simulink model "rake"  (R2017b)
settings: Solver=FixedStepDiscrete  StartTime=0.0  StopTime=0.1  RelTol=1e-3
PreLoadFcn:
  | commwcdmaphlayer_init;
undefined symbols (not defined in the file or in its folder): doppler, totalBitsDelay, trBlkSetSize, tti
libraries: commwcdma_lib x7, commchan3 x3, commrandsrc3 x2, commsink2 x2, commblksprivate x1, commsequence2 x1
Description:
  | WCDMA End-to-End Physical Layer - 3GPP WCDMA FDD (Rel 99) DownLink
settings Model: ExtModeAutoUpdateStatusClock=off  Creator=The MathWorks, Inc.  LastModifiedBy=ericl
settings DataIOCC: SaveFormat=Array  SaveOutput=off  SaveTime=off  SignalLoggingName=wcdmaSigsOut
settings OptimizationCC: BooleanDataType=off  DefaultParameterBehavior=Inlined  InlineInvariantSignals=on  ExpressionDepthLimit=2147483647  InitFltsAndDblsToZero=on  EfficientMapNaN2IntZero=off  LifeSpan=inf
settings DebuggingCC: SaveWithParameterizedLinksMsg=none  UnderspecifiedInitializationDetection=Classic  MergeDetectMultiDrivingBlocksExec=none  CheckExecutionContextPreStartOutputMsg=on  CheckExecutionContextRuntimeOutputMsg=on  SignalResolutionControl=TryResolveAllWithWarning  InheritedTsInSrcMsg=none  MultiTaskDSMMsg=warning  MultiTaskCondExecSysMsg=none  SigSpecEnsureSampleTimeMsg=none  FcnCallInpInsideContextMsg=warning  AllowSymbolicDim=off  StateNameClashWarn=warning  SFUnexpectedBacktrackingDiag=warning  SFNoUnconditionalDefaultTransitionDiag=warning  SFExecutionAtInitializationDiag=none
settings HardwareCC: ProdBitPerPointer=32  ProdBitPerSizeT=32  ProdBitPerPtrDiffT=32  ProdLargestAtomicFloat=None  ProdIntDivRoundTo=Undefined  ProdEndianess=Unspecified  ProdWordSize=32  ProdHWDeviceType=Specified
settings ModelReferenceCC: UpdateModelReferenceTargets=IfOutOfDate  PropagateSignalLabelsOutOfModel=off
settings SFSimCC: SFSimEcho=off  SimCtrlC=off  SimIntegrity=off
settings RTWCC: BuildConfiguration=Faster Runs
settings CodeAppCC: MangleLength=5  StateflowObjectComments=on
settings GRTTargetCC: TargetFcnLib=ansi_tfl_tmw.mat  TargetLangStandard=C89/C90 (ANSI)  GeneratePreprocessorConditionals=Disable all  CombineOutputUpdateFcns=off  GRTInterface=on
settings ConfigComp: CovMetricSettings=dw  CovHtmlReporting=on  CovSaveCumulativeToWorkspaceVar=on  CovSaveSingleToWorkspaceVar=on  CovExternalEMLEnable=off  CovSFcnEnable=off

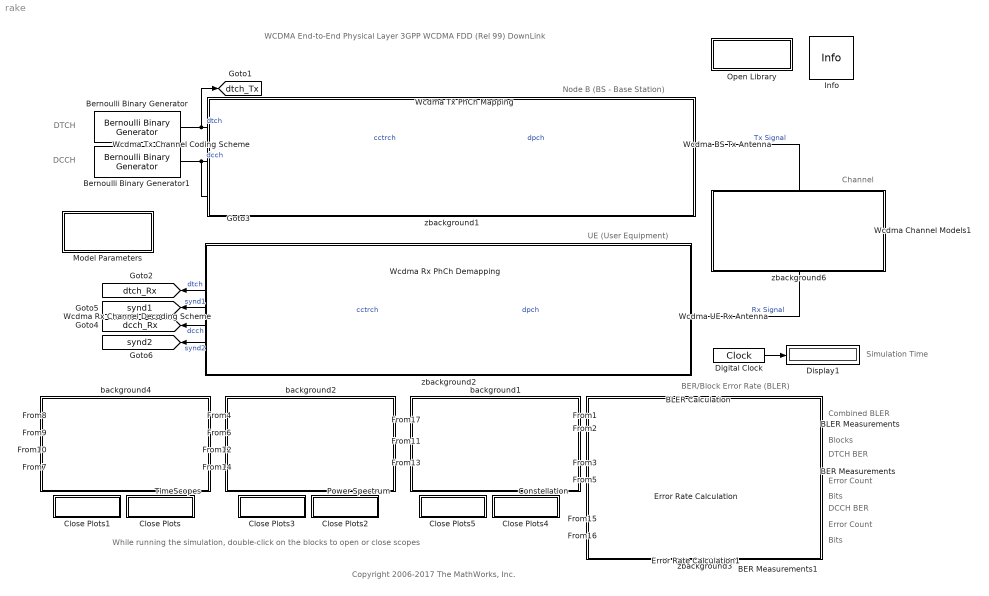
== system rake ==
  note: DTCH
  note: DCCH
  note: DTCH BER
  note: Error Count
  note: Bits
  note: BER/Block Error Rate (BLER)
  note: Combined BLER
  note: Node B (BS - Base Station)
  note: UE (User Equipment)
  note: Channel
  note: WCDMA End-to-End Physical Layer
      | 3GPP WCDMA FDD (Rel 99) DownLink
  note: Blocks
  note: Simulation Time
  note: DCCH BER
  note: Error Count
  note: Bits
  note: While running the simulation, double-click on the blocks to open or close scopes
  note: Copyright 2006-2017 The MathWorks, Inc.
  BER Measurements : Display
  BER Measurements1 : Display
  BLER Calculation : commwcdma_lib/Wcdma Common/BLER Calculation  trBlkSetSize=trBlkSetSize  tti=tti  numBitsDelay=totalBitsDelay
      settings: SourceProductName=Communications System Toolbox  SourceProductBaseCode=CM
  BLER Measurements : Display
  Bernoulli Binary Generator : commrandsrc3/Bernoulli Binary Generator  ProbabilityOfZero=0.5  SeedSource=Parameter  Seed=123456  SampleTime=(tti(1)*1e-3)/trBlkSetSize(1)  SamplesPerFrame=trBlkSetSize(1)  OutputDataType=double  SimulateUsing=Interpreted execution
  Bernoulli Binary Generator1 : commrandsrc3/Bernoulli Binary Generator  ProbabilityOfZero=0.5  SeedSource=Parameter  Seed=123456  SampleTime=(tti(2)*1e-3)/trBlkSetSize(2)  SamplesPerFrame=trBlkSetSize(2)  OutputDataType=double  SimulateUsing=Interpreted execution
  Close Plots : Subsystem
      settings: OpenFcn=|
      | ssName = gcs;
      |   set_param([ssName '/TimeScopes/Real Part'],'Open','off');
      |   set_param([ssName '/TimeScopes/Imag Part'],'Open','off');
      |   set_param([ssName '/TimeScopes/Channel Estimates'],'Open','off');
      | clear ssName;
      mask Display: disp('Close Scopes');
  Close Plots1 : Subsystem
      settings: OpenFcn=|
      | ssName=gcs;
      | set_param([ssName '/TimeScopes/Real Part'],'Open','on');
      |   set_param([ssName '/TimeScopes/Imag Part'],'Open','on');
      |   set_param([ssName '/TimeScopes/Channel Estimates'],'Open','on');
      | clear ssName;
      mask Display: disp('Open Scopes');
  Close Plots2 : Subsystem
      settings: OpenFcn=|
      | set_param([gcs '/Power Spectrum/Before Spreading Spectrum'],'OpenScopeAtSimStart','off');
      |   set_param([gcs '/Power Spectrum/Before Pulse Shaping'],'OpenScopeAtSimStart','off');
      |   set_param([gcs '/Power Spectrum/Tx Signal'],'OpenScopeAtSimStart','off');
      |   set_param([gcs '/Power Spectrum/Rx Signal'],'OpenScopeAtSimStart','off');
      |   sdspfscope2([],[],[],'ScopeUpdate',[gcs '/Power Spectrum/Before Spreading Spectrum'],'CloseFig');
      |   sdspfscope2([],[],[],'ScopeUpdate',[gcs '/Power Spectrum/Before Pulse Shaping'],'CloseFig');
      |   sdspfscope2([],[],[],'ScopeUpdate',[gcs '/Power Spectrum/Tx Signal'],'CloseFig');
      |   sdspfscope2([],[],[],'ScopeUpdate',[gcs '/Power Spectrum/Rx Signal'],'CloseFig');
      mask Display: disp('Close Scopes');
  Close Plots3 : Subsystem
      settings: OpenFcn=|
      | set_param([gcs '/Power Spectrum/Before Spreading Spectrum'],'OpenScopeAtSimStart','on');
      |   set_param([gcs '/Power Spectrum/Before Pulse Shaping'],'OpenScopeAtSimStart','on');
      |   set_param([gcs '/Power Spectrum/Tx Signal'],'OpenScopeAtSimStart','on');
      |   set_param([gcs '/Power Spectrum/Rx Signal'],'OpenScopeAtSimStart','on');
      |   sdspfscope2([],[],[],'ScopeUpdate',[gcs '/Power Spectrum/Before Spreading Spectrum'],'OpenFig');
      |   sdspfscope2([],[],[],'ScopeUpdate',[gcs '/Power Spectrum/Before Pulse Shaping'],'OpenFig');
      |   sdspfscope2([],[],[],'ScopeUpdate',[gcs '/Power Spectrum/Tx Signal'],'OpenFig');
      |   sdspfscope2([],[],[],'ScopeUpdate',[gcs '/Power Spectrum/Rx Signal'],'OpenFig');
      mask Display: disp('Open Scopes');
  Close Plots4 : Subsystem
      settings: OpenFcn=|
      | set_param([bdroot '/Constellation/DPCH_Rx'],'OpenScopeAtSimStart','off');
      | set_param([bdroot '/Constellation/DPCH_Derot'],'OpenScopeAtSimStart','off');
      | set_param([bdroot '/Constellation/DPCH_Comb'],'OpenScopeAtSimStart','off');
      | sdspfscope2([],[],[],'ScopeUpdate',[bdroot '/Constellation/DPCH_Rx'],'CloseFig');
      | sdspfscope2([],[],[],'ScopeUpdate',[bdroot '/Constellation/DPCH_Derot'],'CloseFig');
      | sdspfscope2([],[],[],'ScopeUpdate',[bdroot '/Constellation/DPCH_Comb'],'CloseFig');
      mask Display: disp('Close Scopes');
  Close Plots5 : Subsystem
      settings: OpenFcn=|
      | sdspfscope2([],[],[],'ScopeUpdate',[bdroot '/Constellation/DPCH_Rx'],'OpenFig');
      | sdspfscope2([],[],[],'ScopeUpdate',[bdroot '/Constellation/DPCH_Derot'],'OpenFig');
      | sdspfscope2([],[],[],'ScopeUpdate',[bdroot '/Constellation/DPCH_Comb'],'OpenFig');
      | set_param([bdroot '/Constellation/DPCH_Rx'],'OpenScopeAtSimStart','on');
      | set_param([bdroot '/Constellation/DPCH_Derot'],'OpenScopeAtSimStart','on');
      | set_param([bdroot '/Constellation/DPCH_Comb'],'OpenScopeAtSimStart','on');
      mask Display: disp('Open Scopes');
  Constellation : Subsystem  TreatAsAtomicUnit=on
      mask Display: disp('Scatter\nPlot')
  Digital Clock : DigitalClock  SampleTime=0.001/15
  Display1 : Display
  Error Rate Calculation : commsink2/Error Rate Calculation  N=totalBitsDelay(1)  st_delay=0  cp_mode=Entire frame  subframe=[]  PMode=Port  WsName=ber  RsMode2=off  stop=off  numErr=100  maxBits=1e6
  Error Rate Calculation1 : commsink2/Error Rate Calculation  N=totalBitsDelay(2)  st_delay=0  cp_mode=Entire frame  subframe=[]  PMode=Port  WsName=ber1  RsMode2=off  stop=off  numErr=100  maxBits=1e6
  Info : commblksprivate/Info  SystemSampleTime=-1
      settings: SourceProductName=Communications System Toolbox  SourceProductBaseCode=CM
  Model Parameters : Subsystem  mask(Model Parameters){measurChannel=12.2 Kbps, trBlkSetSize=[3840 100], trBlkSize=[3840 100], tti=[10 40], crcSize=[16 12], errorCorr=[3 2], RMAttribute=[256 256], posTrChMask=Fixed, numPhCH=1, slotFormat=15, powerVector=[-5.5 -10 -15 -12 -12], dpchCode=7, scrCode=[63 0], numTapsRRC=96, numTapsChEst=21, overSampling=8, propConditions=Static - AWGN, snrdB=-3, fingerEnables=4, fingerPhases=[0 260e-9 521e-9 781e-9], fingerPowers=[0 -3 -6 -9], speed=250}
      mask prompts: measurChannel "DL Measurement channels"; trBlkSetSize "Transport block set size:"; trBlkSize "Transport block size:"; tti "TTI (in ms):"; crcSize "CRC Size {24, 16, 12, 8, 0}:"; errorCorr "Error protection {None=0, Conv 1/2=1, Conv 1/3=2, Turbo=3}:"; RMAttribute "Rate matching attribute:"; posTrChMask "Position of TrCH in radio frame:"; numPhCH "Number of PhCH:"; slotFormat "Slot format (0..16):"; powerVector "Power for [DPCH, P-CPICH, PICH, P-CCPCH, SCH] in dB:"; dpchCode "DPCH Code number (0..Spreading Factor -1):"; scrCode "Scrambling code [Scr Code Grup(0..63) Primary Code(0..7)]:"; numTapsRRC "Number of filter taps for RRC:"; numTapsChEst "Number of coefficients for channel estimation filters:"; overSampling "Oversampling factor:"; propConditions "Propagation conditions environments:"; snrdB "SNR (in dB):"; fingerEnables "Number of enable fingers:"; fingerPhases "Relative delay of Rx signals (in s):"; fingerPowers "Average Powers of Rx signals (in dB):"; speed "Speed of Terminal (in Km/h):"
      mask help: Use the following mask to select the different parameters for the simulation.
      mask init:
      | eStr = commwcdmaphlayer_initmask(gcb, 'init', propConditions, powerVector, ...
      |     measurChannel, trBlkSetSize, trBlkSize, tti, crcSize, errorCorr, ...
      |     RMAttribute, posTrChMask, numPhCH, slotFormat, dpchCode, scrCode, ...
      |      numTapsRRC, numTapsChEst, overSampling, snrdB, fingerEnables, ...
      |     fingerPhases, fingerPowers, speed);
      | if(~isempty(eStr.emsg))
      | errordlg(eStr.emsg);
      | end
      | if(~isempty(eStr.emsg_w))
      | disp(eStr.emsg_w);
      | end
      mask Help: helpview(commdhelp);
      mask TypeOptions measurChannel: 12.2 Kbps | 64 Kbps | 144 Kbps | 384 Kbps | User Defined
      mask Callback measurChannel: commwcdmaphlayer_initmask(gcb,'cbMeasurChannel');
      mask TypeOptions posTrChMask: Fixed | Flexible
      mask TypeOptions numPhCH: 1 | 2 | 3
      mask TypeOptions slotFormat: 0 | 1 | 2 | 3 | 4 | 5 | 6 | 7 | 8 | 9 | 10 | 11 | 12 | 13 | 14 | 15 | 16
      mask TypeOptions overSampling: 2 | 4 | 6 | 8 | 10 | 12 | 14 | 16
      mask TypeOptions propConditions: No Channel | Static - AWGN | Multipath Profile - Case 1 | Multipath Profile - Case 2 | Multipath Profile - Case 3 | Multipath Profile - Case 4 | Multipath Profile - Case 5 | Multipath Profile - Case 6 | User Defined
      mask Callback propConditions: commwcdmaphlayer_initmask(gcb, 'cbPropConditions');
      mask TypeOptions fingerEnables: 1 | 2 | 3 | 4
      mask DialogControl Container12 Prompt: Transport Channel
      mask DialogControl TrChInfoTattoo Prompt:
      | Tranport block set size
      | Transport block size
      | TTI (in ms)
      | CRC size
      | Type of error protection
      | Rate matching attribute
      | Position of TrCH in radio frame
      | Number of PhCH
      | Slot format
      mask DialogControl TrChInfoVal Prompt:
      | : [244 100]
      | : [244 100]
      | : [20 40]
      | : [16 12]
      | : [Conv-1/3 Conv-1/3]
      | : [256 256]
      | : Fixed
      | : 1
      | : 11
      mask DialogControl Container13 Prompt: Antenna
      mask DialogControl Container18 Prompt: Channel Model
      mask DialogControl ChMdlInfoTattoo Prompt:
      | Number of enable fingers
      | Relative delay of Rx signals (in s)
      | Average power of Rx signals (in dB)
      | Speed of Terminal (in Km/h)
      mask DialogControl ChMdlInfoVal Prompt:
      | : 2
      | : [0 976e-9]
      | : [0 -10]
      | : 3
      mask Display: disp('Model\nParameters');
  Open Library : Subsystem
      settings: OpenFcn=open('commwcdma_lib');
      mask Display: disp('WCDMA\nLibrary')
  Power Spectrum : Subsystem  TreatAsAtomicUnit=on
      mask Display: disp('Power\nSpectrum')
  TimeScopes : Subsystem  TreatAsAtomicUnit=on
      mask Display: disp('Time\nScopes')
  Wcdma BS Tx Antenna : commwcdma_lib/Wcdma BS Transmitter/Wcdma BS Tx Antenna  slotFormat=slotFormat  dpchCode=dpchCode  scrCode=scrCode  powerVector=powerVector  numTapsRRC=numTapsRRC  overSampling=overSampling  checkparams=off
      settings: SourceProductName=Communications System Toolbox  SourceProductBaseCode=CM
  Wcdma Channel Models1 : Subsystem  Variant=on
      settings: AttributesFormatString=%<BlockChoice>
  Wcdma Rx Channel Decoding Scheme : commwcdma_lib/Wcdma Multiplexing and Channel Coding/Wcdma Rx Channel Decoding Scheme  trBlkSetSize=trBlkSetSize  trBlkSize=trBlkSize  tti=tti  crcSize=crcSize  errorCorr=errorCorr  RMAttribute=RMAttribute  posTrCh=posTrCh  numPhCH=numPhCH  slotFormat=slotFormat  checkParams=off
      settings: SourceProductName=Communications System Toolbox  SourceProductBaseCode=CM
  Wcdma Rx PhCh Demapping : commwcdma_lib/Wcdma Multiplexing and Channel Coding/Wcdma Rx PhCh Demapping  numBitsRF=numBitsRF  numPhCH=numPhCH  slotFormat=slotFormat  checkParams=off
      settings: SourceProductName=Communications System Toolbox  SourceProductBaseCode=CM
  Wcdma Tx PhCh Mapping : commwcdma_lib/Wcdma Multiplexing and Channel Coding/Wcdma Tx PhCh Mapping  numBitsRF=numBitsRF  numPhCH=numPhCH  slotFormat=slotFormat  checkParams=off
      settings: SourceProductName=Communications System Toolbox  SourceProductBaseCode=CM
  Wcdma Tx Channel Coding Scheme : commwcdma_lib/Wcdma Multiplexing and Channel Coding/Wcdma Tx  Channel Coding Scheme  trBlkSetSize=trBlkSetSize  trBlkSize=trBlkSize  tti=tti  crcSize=crcSize  errorCorr=errorCorr  RMAttribute=RMAttribute  posTrCh=posTrCh  numPhCH=numPhCH  slotFormat=slotFormat  checkParams=off
      settings: SourceProductName=Communications System Toolbox  SourceProductBaseCode=CM
  Wcdma UE Rx Antenna : commwcdma_lib/Wcdma UE Receiver/Wcdma UE Rx Antenna  slotFormat=slotFormat  dpchCode=dpchCode  scrCode=scrCode  powerVector=powerVector  snrdB=snrdB  numTapsRRC=numTapsRRC  overSampling=overSampling  fingerEnables=fingerEnables  fingerPhases=fingerPhases  numTapsChEst=numTapsChEst  checkParams=off
      settings: SourceProductName=Communications System Toolbox  SourceProductBaseCode=CM
  background1 : Subsystem
      mask Display: disp('')
  background2 : Subsystem
      mask Display: disp('')
  background4 : Subsystem
      mask Display: disp('')
  zbackground1 : Subsystem  Priority=0
      mask Display: disp('')
  zbackground2 : Subsystem
      mask Display: disp('')
  zbackground3 : Subsystem
      mask Display: disp('')
  zbackground6 : Subsystem
      mask Display: disp('');
  tag scope: dcch_Rx=global, dcch_Tx=global, dtch_Rx=global, dtch_Tx=global, synd1=global, synd2=global
  wires:
  Bernoulli Binary Generator/1 -> [dtch_Tx], Wcdma Tx Channel Coding Scheme/1  "dtch"
  [dtch_Tx] -> Error Rate Calculation/1
  [dtch_Rx] -> Error Rate Calculation/2
  Wcdma Rx Channel Decoding Scheme/1 -> [dtch_Rx]  "dtch"
  Wcdma Rx Channel Decoding Scheme/3 -> [dcch_Rx]  "dcch"
  Wcdma Rx PhCh Demapping/1 -> Wcdma Rx Channel Decoding Scheme/1  "cctrch"
  Wcdma UE Rx Antenna/1 -> Wcdma Rx PhCh Demapping/1  "dpch"
  BLER Calculation/1 -> BLER Measurements/1
  Wcdma Rx Channel Decoding Scheme/2 -> [synd1]  "synd1"
  Wcdma Rx Channel Decoding Scheme/4 -> [synd2]  "synd2"
  [synd1] -> BLER Calculation/1
  [synd2] -> BLER Calculation/2
  Digital Clock/1 -> Display1/1
  Wcdma Tx Channel Coding Scheme/1 -> Wcdma Tx PhCh Mapping/1  "cctrch"
  Wcdma BS Tx Antenna/1 -> Wcdma Channel Models1/1(ChIn)  "Tx Signal"
  Wcdma Channel Models1/1(ChOut) -> Wcdma UE Rx Antenna/1  "Rx Signal"
  Bernoulli Binary Generator1/1 -> Wcdma Tx Channel Coding Scheme/2, [dcch_Tx]  "dcch"
  Wcdma Tx PhCh Mapping/1 -> Wcdma BS Tx Antenna/1  "dpch"
  [dcch_Tx] -> Error Rate Calculation1/1
  [dcch_Rx] -> Error Rate Calculation1/2
  [DPCH_Tx] -> TimeScopes/1(In1)
  [DPCH_Tx_sprd] -> TimeScopes/2(In2)
  [DPCH_Tx_all] -> TimeScopes/3(In3)
  [chEst] -> TimeScopes/4(In5)
  [DPCH_Tx] -> Power Spectrum/1(In1)
  [DPCH_Tx_all] -> Power Spectrum/2(In3)
  [ToChannel] -> Power Spectrum/3(In4)
  [RxSignal] -> Power Spectrum/4(In6)
  [DPCH_Rx] -> Constellation/1(In1)
  [DPCH_Derot] -> Constellation/2(In2)
  [DPCH_Comb] -> Constellation/3(In3)
  Error Rate Calculation/1 -> BER Measurements/1
  Error Rate Calculation1/1 -> BER Measurements1/1

== system rake/Close Plots ==

== system rake/Close Plots1 ==

== system rake/Close Plots2 ==

== system rake/Close Plots3 ==

== system rake/Close Plots4 ==

== system rake/Close Plots5 ==

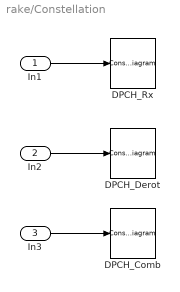
== system rake/Constellation ==
  In1 : Inport
  In2 : Inport  Port=2
  In3 : Inport  Port=3
  DPCH_Comb : ConstellationDiagram  Tag=ScatterPlot
  DPCH_Derot : ConstellationDiagram  Tag=ScatterPlot
  DPCH_Rx : ConstellationDiagram  Tag=ScatterPlot
  wires:
  In1/1 -> DPCH_Rx/1
  In2/1 -> DPCH_Derot/1
  In3/1 -> DPCH_Comb/1

== system rake/Model Parameters ==

== system rake/Open Library ==
  note: This subsystem is intentionally left empty

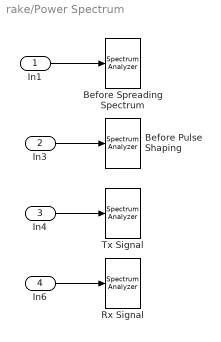
== system rake/Power Spectrum ==
  In1 : Inport
  In3 : Inport  Port=2
  In4 : Inport  Port=3
  In6 : Inport  Port=4
  Before Pulse Shaping : SpectrumAnalyzer
  Before Spreading Spectrum : SpectrumAnalyzer
  Rx Signal : SpectrumAnalyzer
  Tx Signal : SpectrumAnalyzer
  wires:
  In6/1 -> Rx Signal/1
  In4/1 -> Tx Signal/1
  In3/1 -> Before Pulse Shaping/1
  In1/1 -> Before Spreading Spectrum/1

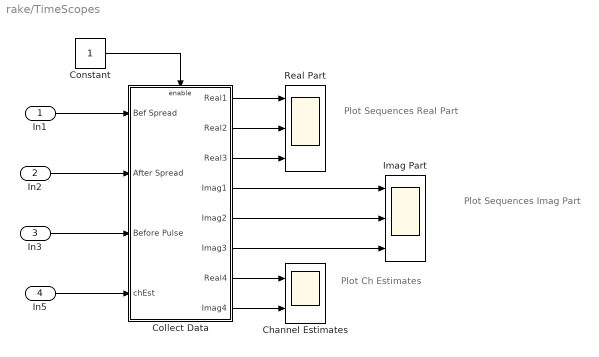
== system rake/TimeScopes ==
  note: Plot Sequences
      | Real Part
  note: Plot Sequences
      | Imag Part
  note: Plot
      | Ch Estimates
  In1 : Inport
  In2 : Inport  Port=2
  In3 : Inport  Port=3
  In5 : Inport  Port=4
  Channel Estimates : Scope  NumInputPorts=2
  Collect Data : Subsystem  TreatAsAtomicUnit=on
  Constant : Constant  VectorParams1D=off  SampleTime=1/15e3
  Imag Part : Scope  NumInputPorts=3
  Real Part : Scope  NumInputPorts=3
  wires:
  Collect Data/8(Imag4) -> Channel Estimates/2
  Collect Data/7(Real4) -> Channel Estimates/1
  Constant/1 -> Collect Data/Enable
  Collect Data/6(Imag3) -> Imag Part/3
  Collect Data/5(Imag2) -> Imag Part/2
  Collect Data/4(Imag1) -> Imag Part/1
  Collect Data/3(Real3) -> Real Part/3
  Collect Data/2(Real2) -> Real Part/2
  Collect Data/1(Real1) -> Real Part/1
  In1/1 -> Collect Data/1(Bef Spread)
  In2/1 -> Collect Data/2(After Spread)
  In3/1 -> Collect Data/3(Before Pulse)
  In5/1 -> Collect Data/4(chEst)

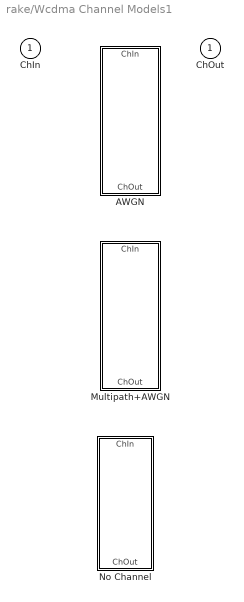
== system rake/Wcdma Channel Models1 ==
  ChIn : Inport
  AWGN : Subsystem  VariantControl=wcdmaChannelID == 2
      mask Display: disp('Wcdma Channel Model:\nAWGN Channel');
  Multipath+AWGN : Subsystem  VariantControl=wcdmaChannelID == 3
      mask Display: disp('Wcdma Channel Model:\nMultipath-AWGN Channel');
  No Channel : Subsystem  VariantControl=wcdmaChannelID == 1
      mask Display: disp('Wcdma Channel Model:\nNo Channel');
  ChOut : Outport

== system rake/background1 ==

== system rake/background2 ==

== system rake/background4 ==

== system rake/zbackground1 ==

== system rake/zbackground2 ==

== system rake/zbackground3 ==

== system rake/zbackground6 ==

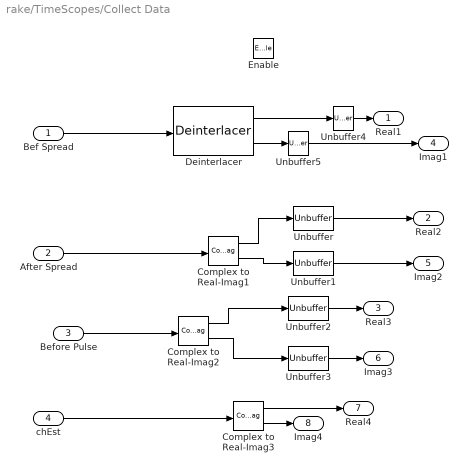
== system rake/TimeScopes/Collect Data ==
  Bef Spread : Inport
  After Spread : Inport  Port=2
  Before Pulse : Inport  Port=3
  chEst : Inport  Port=4
  Enable : EnablePort  PropagateVarSize=During execution
  Complex to Real-Imag1 : ComplexToRealImag
  Complex to Real-Imag2 : ComplexToRealImag
  Complex to Real-Imag3 : ComplexToRealImag
  Deinterlacer : commsequence2/Deinterlacer
      settings: SourceProductName=Communications System Toolbox  SourceProductBaseCode=CM
  Unbuffer{,1..5} (6 alike) : Unbuffer
  Real1 : Outport
  Real2 : Outport  Port=2
  Real3 : Outport  Port=3
  Imag1 : Outport  Port=4
  Imag2 : Outport  Port=5
  Imag3 : Outport  Port=6
  Real4 : Outport  Port=7
  Imag4 : Outport  Port=8
  wires:
  chEst/1 -> Complex to Real-Imag3/1
  Unbuffer5/1 -> Imag1/1
  Unbuffer4/1 -> Real1/1
  Deinterlacer/2 -> Unbuffer5/1
  Deinterlacer/1 -> Unbuffer4/1
  Complex to Real-Imag3/2 -> Imag4/1
  Complex to Real-Imag3/1 -> Real4/1
  Unbuffer3/1 -> Imag3/1
  Unbuffer2/1 -> Real3/1
  Before Pulse/1 -> Complex to Real-Imag2/1
  Complex to Real-Imag2/1 -> Unbuffer2/1
  Complex to Real-Imag2/2 -> Unbuffer3/1
  Complex to Real-Imag1/1 -> Unbuffer/1
  Unbuffer1/1 -> Imag2/1
  Unbuffer/1 -> Real2/1
  Complex to Real-Imag1/2 -> Unbuffer1/1
  After Spread/1 -> Complex to Real-Imag1/1
  Bef Spread/1 -> Deinterlacer/1

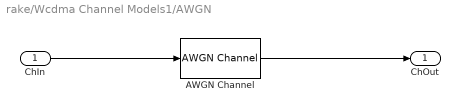
== system rake/Wcdma Channel Models1/AWGN ==
  ChIn : Inport
  AWGN Channel : commchan3/AWGN Channel  InputProcessing=Columns as channels (frame based)  seed=1237  noiseMode="Signal to noise ratio  (Es/No)"  EbNodB=10  EsNodB=snrdB  SNRdB=snrdB  bitsPerSym=1  Ps=1  Tsym=1/3.84e6  variance=1
  ChOut : Outport
  wires:
  AWGN Channel/1 -> ChOut/1
  ChIn/1 -> AWGN Channel/1

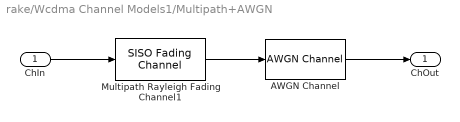
== system rake/Wcdma Channel Models1/Multipath+AWGN ==
  ChIn : Inport
  AWGN Channel : commchan3/AWGN Channel  InputProcessing=Columns as channels (frame based)  seed=1237  noiseMode="Signal to noise ratio  (Es/No)"  EbNodB=10  EsNodB=snrdB  SNRdB=snrdB  bitsPerSym=1  Ps=1  Tsym=1/3.84e6  variance=1
  Multipath Rayleigh Fading Channel1 : commchan3/SISO Fading Channel  PathDelays=fingerPhases  AveragePathGains=fingerPowers  NormalizePathGains=off  FadingDistribution=Rayleigh  KFactor=3  DirectPathDopplerShift=0  DirectPathInitialPhase=0  MaximumDopplerShift=dopplerFreq  DopplerSpectrum=doppler('Jakes')  RandomStream=mt19937ar with seed  RandomNumGenerator=mt19937ar  Seed=12345  PathGainsOutputPort=off  ChannelFilterDelayOutputPort=off  SimulateUsing=Interpreted execution  Visualization=Off  PathsForDopplerDisplay=1  SamplesToDisplay=25%
      settings: SourceProductName=Communications System Toolbox
  ChOut : Outport
  wires:
  Multipath Rayleigh Fading Channel1/1 -> AWGN Channel/1
  ChIn/1 -> Multipath Rayleigh Fading Channel1/1
  AWGN Channel/1 -> ChOut/1

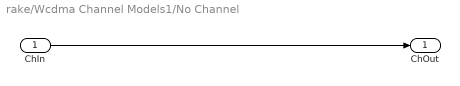
== system rake/Wcdma Channel Models1/No Channel ==
  ChIn : Inport
  ChOut : Outport
  wires:
  ChIn/1 -> ChOut/1
